simulink model "process_sensors"  (R2025b)
settings: configuration reference "MCConfiguration" (kept outside this file)
undefined symbols (not defined in the file): motorsensors, Ts_ControlFOC
libraries: dspsigops x2, mcbhdlpositiondecoderlib x1
settings Model: DataDictionary=embeddedBoard_common.sldd  Creator=rpumpo  LastModifiedBy=rpumpo
settings ConfigSetRef: SourceName=MCConfiguration

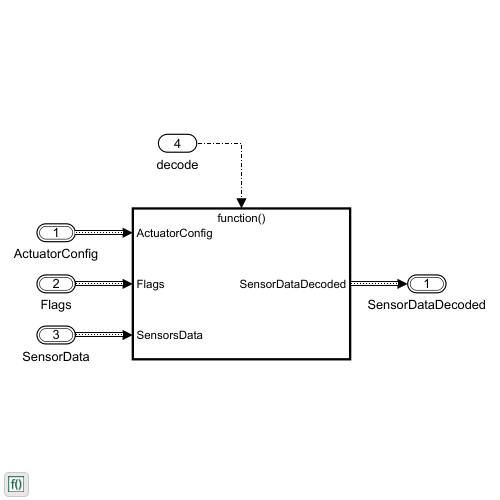
[thumbnail: Simulink's stored preview of the top-level diagram]
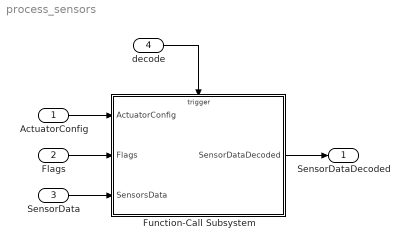
== system process_sensors ==
  ActuatorConfig : Inport  OutDataTypeStr=Bus: ActuatorConfiguration  BusOutputAsStruct=on
  Flags : Inport  Port=2  OutDataTypeStr=Bus: Flags  BusOutputAsStruct=on
  SensorData : Inport  Port=3  OutDataTypeStr=Bus: SensorsData  BusOutputAsStruct=on
  decode : Inport  Port=4  SampleTime=Ts_ControlFOC  OutputFunctionCall=on
  Function-Call Subsystem : Subsystem  TreatAsAtomicUnit=on
  SensorDataDecoded : Outport  OutDataTypeStr=Bus: SensorsData  BusOutputAsStruct=on
  wires:
  Function-Call Subsystem/1(SensorDataDecoded) -> SensorDataDecoded/1
  ActuatorConfig/1 -> Function-Call Subsystem/1(ActuatorConfig)
  Flags/1 -> Function-Call Subsystem/2(Flags)
  SensorData/1 -> Function-Call Subsystem/3(SensorsData)
  decode/1 -> Function-Call Subsystem/Trigger

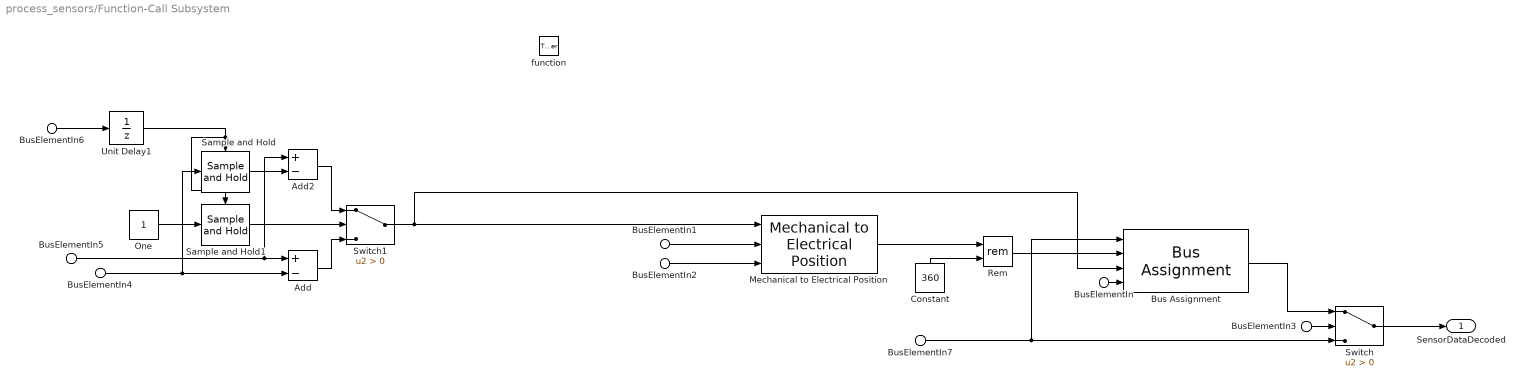
== system process_sensors/Function-Call Subsystem ==
  BusElementIn3 : Inport  PortName=ActuatorConfig  Element=motor.externals.has_quadrature_encoder
  BusElementIn1 : Inport  PortName=ActuatorConfig  Element=motor.externals.pole_pairs
  BusElementIn2 : Inport  PortName=ActuatorConfig  Element=motor.externals.rotor_index_offset
  BusElementIn6 : Inport  Port=2  PortName=Flags  Element=calibration_done
  BusElementIn7 : Inport  Port=3  PortName=SensorsData
  BusElementIn5 : Inport  Description=Counter of the QENC  Port=3  PortName=SensorsData  Element=motorsensors.qencoder.counter
  BusElementIn4 : Inport  Description=Last QENC count where the index has been detected  Port=3  PortName=SensorsData  Element=motorsensors.qencoder.Idx_counter
  BusElementIn : Inport  Port=3  PortName=SensorsData  Element=motorsensors.Iabc
  function : TriggerPort  TriggerType=function-call  VariantControl=(inherit)
  Add : Sum  Inputs=+-
  Add2 : Sum  Inputs=+-
  Bus Assignment : BusAssignment  AssignedSignals=motorsensors.electrical_angle,motorsensors.qencoder.rotor_angle,motorsensors.Iabc
  Constant : Constant  Value=360  OutDataTypeStr=single
  Mechanical to Electrical Position : mcbhdlpositiondecoderlib/Mechanical to Electrical Position  PolePairsInputType=Input port  NrPP=4  selectedRange=Degrees  MechOfstInputType=Input port  mechOffsetIn=0  maxAngleIn=360  InputDataType=single  VariantSelect=floating-point
      settings: LibrarySourceBlock=mcbhdllib/Sensor Decoders/Mechanical to Electrical Position
  One : Constant  OutDataTypeStr=Inherit: Inherit via back propagation
  Rem : Math  Operator=rem
  Sample and Hold : dspsigops/Sample and Hold  trig=Rising edge  initCond=0  latchinput=off
  Sample and Hold1 : dspsigops/Sample and Hold  trig=Rising edge  initCond=0  latchinput=off
  Switch : Switch  Criteria=u2 > Threshold  SaturateOnIntegerOverflow=off  InputSameDT=off
  Switch1 : Switch  Criteria=u2 > Threshold  SaturateOnIntegerOverflow=off  InputSameDT=off
  Unit Delay1 : UnitDelay  SampleTime=-1  HasFrameUpgradeWarning=on
  SensorDataDecoded : Outport  OutDataTypeStr=Bus: SensorsData  BusOutputAsStruct=on
  wires:
  Rem/1 -> Bus Assignment/2
  One/1 -> Sample and Hold1/1
  Switch1/1 -> Mechanical to Electrical Position/1, Bus Assignment/3
  Switch/1 -> SensorDataDecoded/1
  Add2/1 -> Switch1/1
  BusElementIn3/1 -> Switch/2
  Unit Delay1/1 -> Sample and Hold1/Trigger, Sample and Hold/Trigger
  Mechanical to Electrical Position/1 -> Rem/1
  Constant/1 -> Rem/2
  Sample and Hold1/1 -> Switch1/2
  Sample and Hold/1 -> Add2/2
  BusElementIn6/1 -> Unit Delay1/1
  Add/1 -> Switch1/3
  Bus Assignment/1 -> Switch/1
  BusElementIn2/1 -> Mechanical to Electrical Position/3
  BusElementIn1/1 -> Mechanical to Electrical Position/2
  BusElementIn7/1 -> Bus Assignment/1, Switch/3
  BusElementIn/1 -> Bus Assignment/4
  BusElementIn4/1 -> Sample and Hold/1, Add/2
  BusElementIn5/1 -> Add2/1, Add/1
